simulink model "stellaris_lp_irreceive_servo"  (R2017a)
settings: Solver=FixedStepDiscrete  StartTime=0.0  StopTime=10.0  FixedStep=ts  RelTol=1e-3
undefined symbols (not defined in the file or in its folder): ts
libraries: stellaris_lp_lib x5, simulink x3
settings Model: ExtModeTrigDuration=2  Creator=peselnikmg  LastModifiedBy=Nilim
settings DataIOCC: LimitDataPoints=on  SaveFormat=Array  SignalLoggingSaveFormat=ModelDataLogs  ReturnWorkspaceOutputs=on
settings OptimizationCC: UseDivisionForNetSlopeComputation=on  UseFloatMulNetSlope=on  UseSpecifiedMinMax=on  PassReuseOutputArgsAs=Individual arguments  ExpressionDepthLimit=2147483647  ZeroExternalMemoryAtStartup=off  ZeroInternalMemoryAtStartup=off  NoFixptDivByZeroProtection=on  EfficientFloat2IntCast=on  LifeSpan=inf  MaxStackSize=64  OptimizeBlockOrder=speed
settings DebuggingCC: ReadBeforeWriteMsg=DisableAll  WriteAfterWriteMsg=DisableAll  WriteAfterReadMsg=DisableAll  MultiTaskDSMMsg=none  IntegerOverflowMsg=error  ParameterTunabilityLossMsg=error  AssertControl=DisableAll  StateNameClashWarn=warning  NonBusSignalsTreatedAsBus=error  SFInvalidInputDataAccessInChartInitDiag=error  SFTransitionOutsideNaturalParentDiag=error  SFUnreachableExecutionPathDiag=error  SFUndirectedBroadcastEventsDiag=error  SFExecutionAtInitializationDiag=none  IntegerSaturationMsg=error
settings HardwareCC: ProdBitPerPointer=32  ProdBitPerSizeT=32  ProdBitPerPtrDiffT=32  ProdLargestAtomicInteger=Long  ProdLargestAtomicFloat=Double  ProdWordSize=32  ProdHWDeviceType=ARM Compatible->ARM Cortex
settings ModelReferenceCC: UpdateModelReferenceTargets=IfOutOfDate  PropagateSignalLabelsOutOfModel=off
settings SFSimCC: SFSimEcho=off  MATLABDynamicMemAlloc=off
settings RTWCC: SystemTargetFile=ert.tlc  HardwareBoard=Tiva TM4C123G Launchpad  TLCOptions=-aInlineSetEventsForThisBaseRateFcn=TLC_FALSE -aSuppressMultiTaskScheduler=TLC_FALSE -aRateBasedStepFcn=1  TemplateMakefile=ert_default_tmf  Description=Embedded Coder  GenerateReport=on  RTWVerbose=off  Toolchain=Texas Instruments Code Composer Studio (Tiva)  BuildConfiguration=Faster Runs  IncludeHyperlinkInReport=on  LaunchReport=on  GenerateTraceInfo=on  GenerateTraceReport=on  GenerateTraceReportSl=on  GenerateTraceReportSf=on  GenerateTraceReportEml=on
settings CodeAppCC: ForceParamTrailComments=on  IgnoreCustomStorageClasses=off  OperatorAnnotations=on  SimulinkDataObjDesc=on  SFDataObjDesc=on  MATLABFcnDesc=on  CustomSymbolStrType=$N$R$M  InsertBlockDesc=on  MATLABSourceComments=on  EnableCustomComments=on  ReqsInCode=on
settings ERTTargetCC: UtilityFuncGeneration=Shared location  CombineSignalStateStructs=on  SuppressErrorStatus=on  SupportNonFinite=off  ParenthesesLevel=Maximum  CastingMode=Standards  EnableSignedLeftShifts=off  EnableSignedRightShifts=off
settings ConfigComp: CovMetricSettings=dw  CovHtmlReporting=on  CovSaveCumulativeToWorkspaceVar=on  CovSaveSingleToWorkspaceVar=on  CovExternalEMLEnable=off

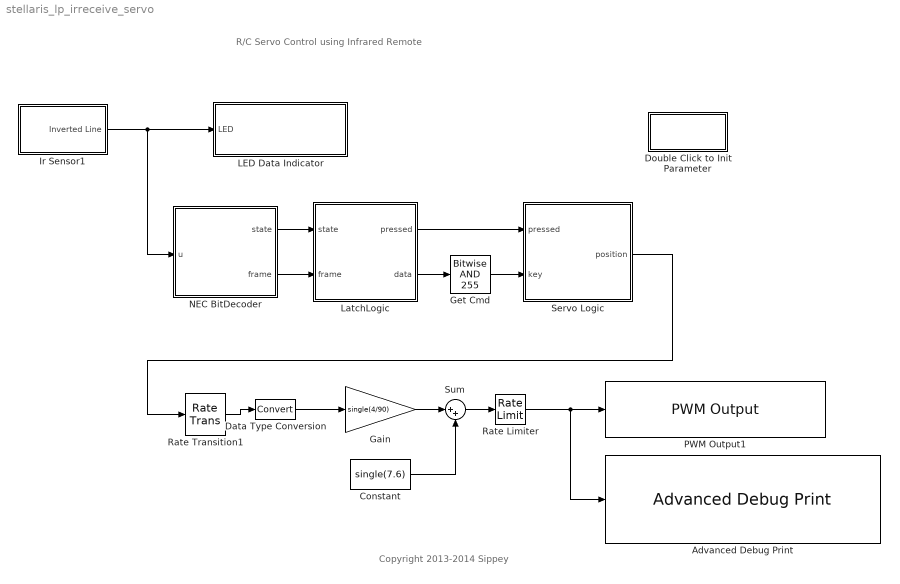
== system stellaris_lp_irreceive_servo ==
  note: R/C Servo Control using Infrared Remote
  note: Copyright 2013-2014 Sippey
  Advanced Debug Print : stellaris_lp_lib/Debug/Advanced Debug Print  types={'single'}  fmt='Position=%hf\r\n'  sample_time=0.02
      settings: SourceProductName=Run on Stellaris LaunchPad
  Constant : Constant  Value=single(7.6)
  Data Type Conversion : DataTypeConversion
  Double Click to Init Parameter : Subsystem
      settings: OpenFcn=ts=0.0001;
      mask Display: fprintf('Double-click');
  Gain : Gain  Gain=single(4/90)
  Get Cmd : simulink/Logic and Bit Operations/Bitwise Operator  logicop=AND  UseBitMask=on  BitMask=255  BitMaskRealWorld=Stored Integer
  Ir Sensor1 : Subsystem
  LED Data Indicator : Subsystem
  LatchLogic : Stateflow chart  TreatAsAtomicUnit=on
  NEC BitDecoder : Stateflow chart  TreatAsAtomicUnit=on
  PWM Output1 : stellaris_lp_lib/PWM/PWM Output  ch="1    PC4"  invert=off  freq=50  sample_time=0.02
      settings: SourceProductName=Run on Stellaris LaunchPad
  Rate Limiter : RateLimiter  RisingSlewLimit=single(8)  FallingSlewLimit=single(-8)  SampleTimeMode=inherited  InitialCondition=single(7.6)
  Rate Transition1 : RateTransition  OutPortSampleTime=0.02
  Servo Logic : Stateflow chart  TreatAsAtomicUnit=on
  Sum : Sum  Inputs=|++
  wires:
  Ir Sensor1/1(Inverted Line) -> NEC BitDecoder/1(u), LED Data Indicator/1(LED)
  Get Cmd/1 -> Servo Logic/2(key)
  Rate Transition1/1 -> Data Type Conversion/1
  Servo Logic/1(position) -> Rate Transition1/1
  Sum/1 -> Rate Limiter/1
  Data Type Conversion/1 -> Gain/1
  Gain/1 -> Sum/1
  Constant/1 -> Sum/2
  Rate Limiter/1 -> PWM Output1/1, Advanced Debug Print/1
  NEC BitDecoder/1(state) -> LatchLogic/1(state)
  NEC BitDecoder/2(frame) -> LatchLogic/2(frame)
  LatchLogic/2(data) -> Get Cmd/1
  LatchLogic/1(pressed) -> Servo Logic/1(pressed)

== system stellaris_lp_irreceive_servo/Double Click to Init Parameter ==

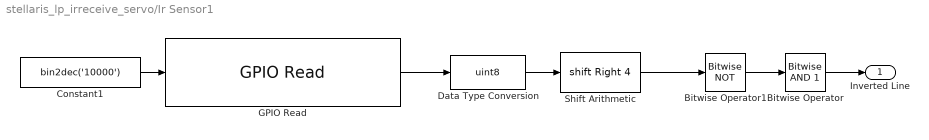
== system stellaris_lp_irreceive_servo/Ir Sensor1 ==
  Bitwise Operator : simulink/Logic and Bit Operations/Bitwise Operator  logicop=AND  UseBitMask=on  BitMask=1  BitMaskRealWorld=Stored Integer
  Bitwise Operator1 : simulink/Logic and Bit Operations/Bitwise Operator  logicop=NOT  UseBitMask=off  BitMask=1  BitMaskRealWorld=Stored Integer
  Constant1 : Constant  Value=bin2dec('10000')  OutDataTypeStr=Inherit: Inherit via back propagation
  Data Type Conversion : DataTypeConversion  OutDataTypeStr=uint8  SampleTime=ts
  GPIO Read : stellaris_lp_lib/GPIO/GPIO Read  GPIO_PORTX_BASE=GPIO_PORTF_BASE  SampleTime=-1
      settings: SourceProductName=Run on Stellaris LaunchPad
  Shift Arithmetic : ArithShift  BitShiftNumber=4  BitShiftDirection=Right
  Inverted Line : Outport
  wires:
  Constant1/1 -> GPIO Read/1
  Shift Arithmetic/1 -> Bitwise Operator1/1
  GPIO Read/1 -> Data Type Conversion/1
  Bitwise Operator1/1 -> Bitwise Operator/1
  Bitwise Operator/1 -> Inverted Line/1
  Data Type Conversion/1 -> Shift Arithmetic/1

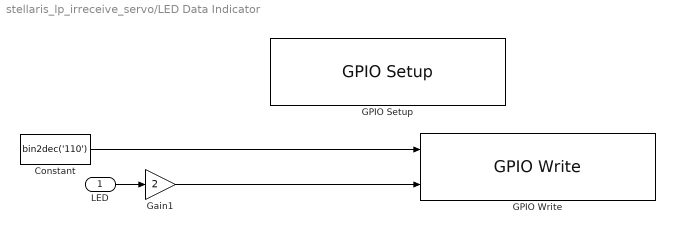
== system stellaris_lp_irreceive_servo/LED Data Indicator ==
  LED : Inport
  Constant : Constant  Value=bin2dec('110')  OutDataTypeStr=Inherit: Inherit via back propagation
  GPIO Setup : stellaris_lp_lib/GPIO/GPIO Setup  GPIO_PORTX_BASE=GPIO_PORTF_BASE  PinsOutput_0=Input  PinsOutput_1=Output  PinsOutput_2=Output  PinsOutput_3=Output  PinsOutput_4=Input  PinsOutput_5=Input  PinsOutput_6=Input  PinsOutput_7=Input
      settings: SourceProductName=Run on Stellaris LaunchPad
  GPIO Write : stellaris_lp_lib/GPIO/GPIO Write  GPIO_PORTX_BASE=GPIO_PORTF_BASE  SampleTime=-1
      settings: SourceProductName=Run on Stellaris LaunchPad
  Gain1 : Gain  Gain=2  OutDataTypeStr=Inherit: Inherit via back propagation
  wires:
  Constant/1 -> GPIO Write/1
  Gain1/1 -> GPIO Write/2
  LED/1 -> Gain1/1

== stateflow chart stellaris_lp_irreceive_servo/LatchLogic ==
  state NotPressed
    pressed=0;
    data=0;
  state Pressed
    pressed=1;
  note: If repeat stub is seen, the bit decoder will go
      | to the BitDecoded state once and then timeout.
      | Reset the temporal logic at this time.
  note: timeout after 125ms
      | if a repeat stub have
      | not show up yet
  (default) -> NotPressed
  NotPressed -> Pressed : [state==1]{data=frame;}
  Pressed -> Pressed [order 2] : [state==-4]
  Pressed -> NotPressed [order 1] : after(0.125,sec)
  data: state input int32 =0; frame input int32; pressed output int32; data output int32

== stateflow chart stellaris_lp_irreceive_servo/Servo Logic ==
  state Pressed
    position=satu_90(position+delta);
  state Reset
    delta=0;
  (default) -> Reset
  (junction 184) -> Pressed [order 4] : [key==240]{delta=-1;}
  Pressed -> Pressed [order 2] : after(0.1,sec)[pressed==1]
  Reset -> (junction 184) [order 1] : [pressed==1]
  (junction 184) -> Pressed [order 1] : [key==200]{delta=1;}
  (junction 184) -> Pressed [order 3] : [key==136]{delta=10;}
  (junction 184) -> Pressed [order 2] : [key==168]{delta=-10;}
  Reset -> Reset [order 2] : [key==84]
  Pressed -> Reset [order 1] : [pressed==0]
  data: u function_input double; y function_output double; pressed input int32 =0; key input int32; position output int32; delta local int32
  function y=satu_90(u):
    | function y=satu_90(u)
    | if u>90
    |     y=90;
    | elseif u<-90;
    |     y=-90;
    | else
    |     y=u;
    | end

== stateflow chart stellaris_lp_irreceive_servo/NEC BitDecoder ==
  note: bit detection timeout 10ms
  note: bit '0': 562.5µs space
      | bit '1': 1.6875ms  space
      | Threshold set to 1ms
  note: invalid start bit
  note: 9ms start pulse
      | set 8ms as threshold
  state StartSym
    state = -2;
  state BitWait
    state= -3;
  state Idle
    state = -1;
    frame=0;
  state BitDecoded
    state=-4;
  state OutStage
    state=1;
  note: output trigger
      | valid for one tick
  note: space between start bit and first data
      | pulse is 4.5ms and will be decoded
      | as a '1' bit, so one more bit to decode.
  BitWait -> Idle [order 3] : after(10e-3,sec)
  (default) -> Idle
  StartSym -> BitWait [order 1] : after(8e-3,sec)
      | [u==0]
      | {nb=0;frame=0;}
  StartSym -> Idle [order 2] : before(8e-3,sec)[u==0]
  BitWait -> BitDecoded [order 2] : after(1e-3,sec)[u==1]{frame=2*frame+1;}
  BitWait -> BitDecoded [order 4] : before(1e-3,sec)[u==1]{frame=2*frame;}
  Idle -> StartSym : [u==1]
  BitDecoded -> BitWait : [u==0]{nb=nb+1;}
  OutStage -> Idle
  BitWait -> OutStage [order 1] : [nb>=25]
  data: u input; state output int32 =0; nb local int32; frame output int32
